simulink model "Sensor_Models"  (R2025b)
settings: Solver=VariableStepAuto  StartTime=0.0  StopTime=10.0  RelTol=1e-3
undefined symbols (not defined in the file or in its folder): constantsASTRA, dt, dt_SIM, IMU_Rate, magDistMatrix
libraries: aerolibnav x2, simulink x1
settings Model: Creator=andrew  LastModifiedBy=andrew

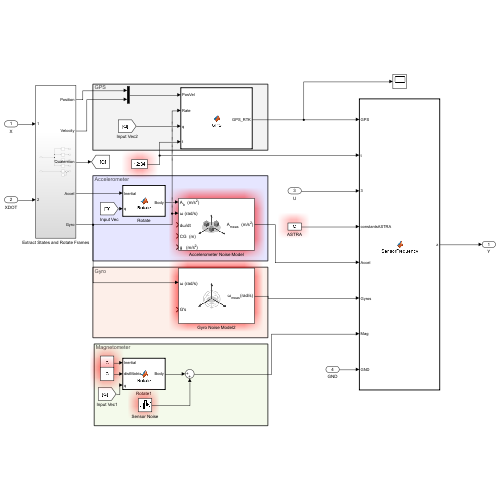
[thumbnail: Simulink's stored preview of the top-level diagram]
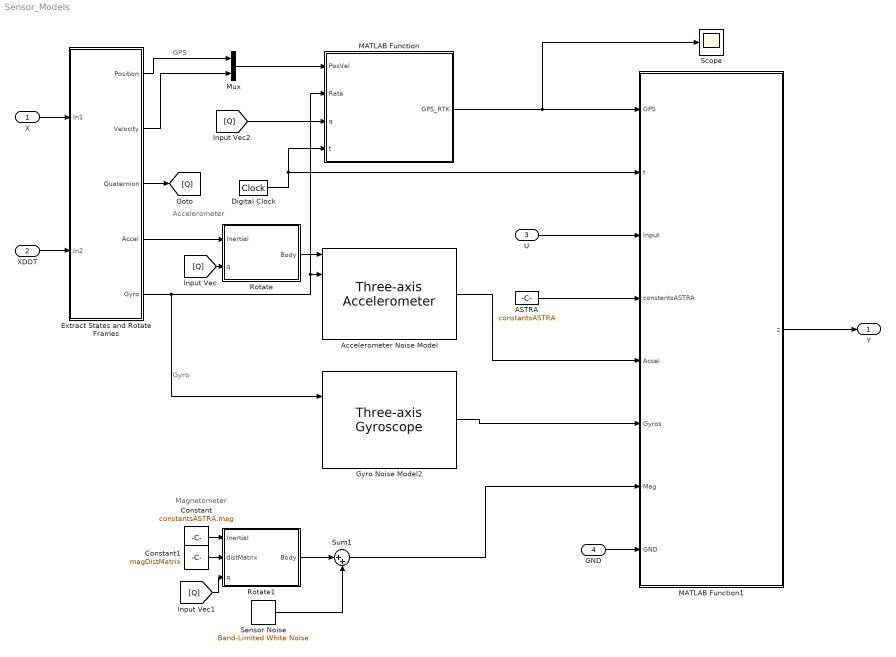
== system Sensor_Models ==
  note: Accelerometer
  note: Gyro
  note: Magnetometer
  note: GPS
  X : Inport
  XDOT : Inport  Port=2
  U : Inport  Port=3
  GND : Inport  Port=4
  ASTRA : Constant  Value=constantsASTRA  OutDataTypeStr=Bus: slBus1
  Accelerometer Noise Model : aerolibnav/Three-axis Accelerometer  units=Metric (MKS)  acc=[0 0 0.15]  gtype=on  dtype_a=on  w_a=190  z_a=0.707  a_sf_cc=eye(3)  a_bias=accelBias  a_Ts=1 / IMU_Rate  a_rand=on  a_seeds=[23093 23094 23095]  a_pow=ones(1,3) * 0.008^2 * 1 / IMU_Rate  a_sat="[-inf  -inf  -inf  inf inf inf]"
  Constant : Constant  Value=constantsASTRA.mag
  Constant1 : Constant  Value=magDistMatrix
  Digital Clock : DigitalClock  SampleTime=dt_SIM
  Extract States and Rotate Frames : Subsystem
  Gyro Noise Model2 : aerolibnav/Three-axis Gyroscope  dtype_g=on  w_g=190  z_g=0.707  g_sf_cc=eye(3)  g_bias=gyroBias  g_sen=0  g_Ts=1 / IMU_Rate  g_rand=on  g_seeds=[23093 23094 23095]  g_pow=ones(1,3) * 0.003^2 * dt  g_sat="[-inf  -inf  -inf  inf inf inf]"
  MATLAB Function : MATLAB Function  TreatAsAtomicUnit=on
  MATLAB Function1 : MATLAB Function  TreatAsAtomicUnit=on
  Mux : Mux  Inputs=2
  Rotate : MATLAB Function  TreatAsAtomicUnit=on
  Rotate1 : MATLAB Function  TreatAsAtomicUnit=on
  Scope : Scope
      settings: ActiveDisplayYMinimum=-1  ActiveDisplayYMaximum=1  DataLoggingVariableName=ScopeData10
  Sensor Noise : simulink/Sources/Band-Limited White Noise  Cov=(4E-4)^2  Ts=dt_SIM  seed=[23341,23342,23343]
  Sum1 : Sum  Inputs=|++
  Y : Outport
  wires:
  Extract States and Rotate Frames/5(Gyro) -> Accelerometer Noise Model/2, MATLAB Function/2(Rate), Gyro Noise Model2/1
  Constant/1 -> Rotate1/1(Inertial)
  U/1 -> MATLAB Function1/3(Input)
  Gyro Noise Model2/1 -> MATLAB Function1/6(Gyros)
  Mux/1 -> MATLAB Function/1(PosVel)
  Extract States and Rotate Frames/1(Position) -> Mux/1
  Extract States and Rotate Frames/2(Velocity) -> Mux/2
  GND/1 -> MATLAB Function1/8(GND)
  Extract States and Rotate Frames/3(Quaternion) -> [Q]
  Rotate/1(Body) -> Accelerometer Noise Model/1
  X/1 -> Extract States and Rotate Frames/1(In1)
  MATLAB Function/1(GPS_RTK) -> Scope/1, MATLAB Function1/1(GPS)
  Constant1/1 -> Rotate1/2(distMatrix)
  ASTRA/1 -> MATLAB Function1/4(constantsASTRA)
  Accelerometer Noise Model/1 -> MATLAB Function1/5(Accel)
  Sum1/1 -> MATLAB Function1/7(Mag)
  MATLAB Function1/1(z) -> Y/1
  Sensor Noise/1 -> Sum1/2
  [Q] -> Rotate/2(q)
  [Q] -> Rotate1/3(q)
  [Q] -> MATLAB Function/3(q)
  Digital Clock/1 -> MATLAB Function/4(t), MATLAB Function1/2(t)
  XDOT/1 -> Extract States and Rotate Frames/2(In2)
  Extract States and Rotate Frames/4(Accel) -> Rotate/1(Inertial)
  Rotate1/1(Body) -> Sum1/1

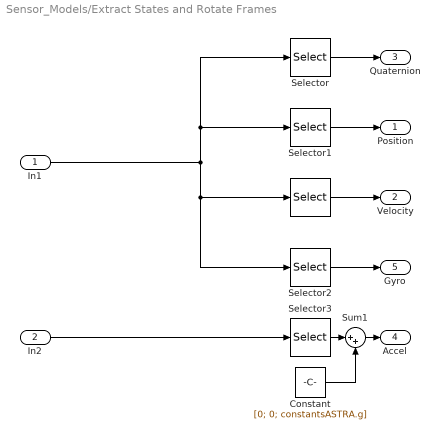
== system Sensor_Models/Extract States and Rotate Frames ==
  In1 : Inport
  In2 : Inport  Port=2
  "  " : Selector  InputPortWidth=16  IndexOptions=Index vector (dialog)  Indices=[8:10]  OutputSizes=1
  Constant : Constant  Value=[0; 0; constantsASTRA.g]
  Selector : Selector  InputPortWidth=16  IndexOptions=Index vector (dialog)  Indices=[1:4]  OutputSizes=1
  Selector1 : Selector  InputPortWidth=16  IndexOptions=Index vector (dialog)  Indices=[5:7]  OutputSizes=1
  Selector2 : Selector  InputPortWidth=16  IndexOptions=Index vector (dialog)  Indices=[11:13]  OutputSizes=1
  Selector3 : Selector  InputPortWidth=16  IndexOptions=Index vector (dialog)  Indices=[8:10]  OutputSizes=1
  Sum1 : Sum  Inputs=|++
  Position : Outport
  Velocity : Outport  Port=2
  Quaternion : Outport  Port=3
  Accel : Outport  Port=4
  Gyro : Outport  Port=5
  wires:
  Selector/1 -> Quaternion/1
  Selector1/1 -> Position/1
  "  "/1 -> Velocity/1
  Selector2/1 -> Gyro/1
  Selector3/1 -> Sum1/1
  Sum1/1 -> Accel/1
  Constant/1 -> Sum1/2
  In1/1 -> Selector1/1, Selector/1, Selector2/1, "  "/1
  In2/1 -> Selector3/1

== matlab function Sensor_Models/Rotate ==
  data: Inertial input; Body output; q input
function Body = Rotate(Inertial, q)
Body = quatRot(q) * Inertial;

== matlab function Sensor_Models/Rotate1 ==
  data: Inertial input; distMatrix input; Body output; q input
function Body = Rotate(Inertial, distMatrix, q)
Body = quatRot(q) * (distMatrix * Inertial + 0.05 * ones(3,1));

== matlab function Sensor_Models/MATLAB Function ==
  data: PosVel input; Rate input; q input; GPS_RTK output; t input
function GPS_RTK = GPS(PosVel, Rate, q, t)

R_b2i = quatRot(q)';
GPS_RTK = GPS_Sim(PosVel, Rate, R_b2i, t);

== matlab function Sensor_Models/MATLAB Function1 ==
  data: GPS input; t input; Input input; constantsASTRA input; Accel input; z output; Gyros input; Mag input; GND input
function z = SensorFrequency(GPS, t, Input, constantsASTRA, Accel, Gyros, Mag, GND)
%% Add Thrust Varying Oscillation
persistent phase lastT
if isempty(phase)
    phase = 0;
    lastT = 0;
end
dt = t - lastT;
lastT = t;

% Thrust vibration generator
Track = [1.3525    42.6278];
THRUST = Input(3) / constantsASTRA.MaxT * 100;
w = 2 * pi * (Track(1) * THRUST + Track(2) + 1 * randn());
phase = phase + w * dt;
MaxAmplAccel = 7;
MaxAmplGyro = 0.2;
Accel = Accel + MaxAmplAccel * THRUST / 100 * sin(phase) * (1 - GND);
Gyros = Gyros + MaxAmplGyro * THRUST / 100 * sin(phase) * (1 - GND);
z = [Accel; Gyros; Mag; GPS];
